simulink model "simulazione_stretch"  (R2024a)
settings: Solver=FixedStepAuto  StartTime=0.0  StopTime=19  FixedStep=0.2  RelTol=1e-3
libraries: robotcorelib x1, robotmaniplib x1
settings Model: Creator=LAIR  LastModifiedBy=LAIR
settings RTWCC: GPUComputeCapability=3.5

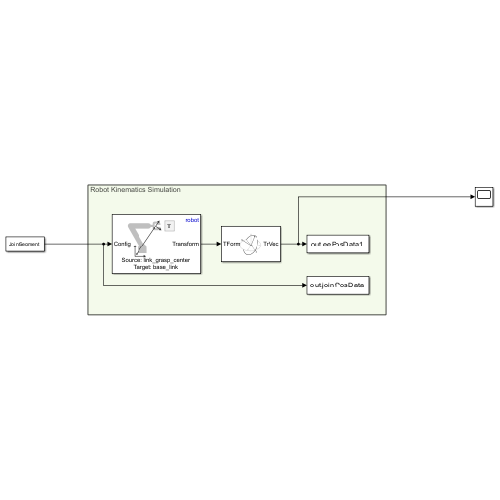
[thumbnail: Simulink's stored preview of the top-level diagram]
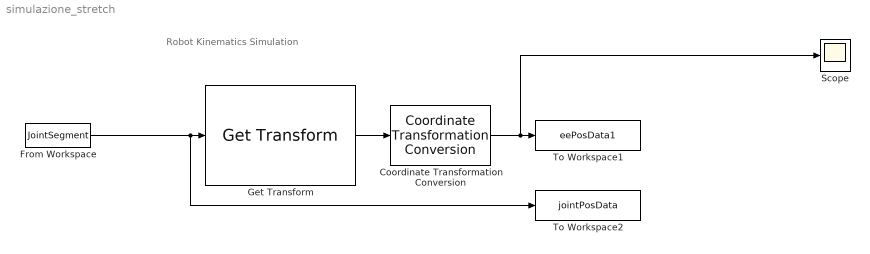
== system simulazione_stretch ==
  note: Robot Kinematics Simulation
  Coordinate Transformation Conversion : robotcorelib/Coordinate Transformation Conversion  InputRepresentation=Homogeneous Transformation  InputEulerSequence=ZYX  ShowTrVecInputPort=on  OutputRepresentation=Translation Vector  OutputEulerSequence=ZYX  ShowTrVecOutputPort=on  SimulateUsing=Interpreted execution
  From Workspace : FromWorkspace  VariableName=JointSegment
  Get Transform : robotmaniplib/Get Transform  RigidBodyTree=robot  SourceBody=link_grasp_center  TargetBody=base_link  SimulateUsing=Interpreted execution
  Scope : Scope
  To Workspace1 : ToWorkspace  VariableName=eePosData1  SaveFormat=Timeseries  SampleTime=-1
  To Workspace2 : ToWorkspace  VariableName=jointPosData  SaveFormat=Timeseries  SampleTime=-1
  wires:
  Get Transform/1 -> Coordinate Transformation Conversion/1
  Coordinate Transformation Conversion/1 -> Scope/1, To Workspace1/1
  From Workspace/1 -> To Workspace2/1, Get Transform/1
